simulink model "S7_Legacy_HotStart_Average_Plant"  (R2024b)
settings: Solver=ode15s  StartTime=0.0  StopTime=10  FixedStep=4e-6  MaxStep=1e-4  RelTol=1e-5  EnableMultiTasking=on
InitFcn:
  | s7SourceDir='D:\博士工作\论文工作\（1）构网型风电机组\构网型风电机组\5MW_Ideal\CurrentModel_Idealized';
  | dtime=4e-6;
  | Ts_step=1e-6;
  | run(fullfile(s7SourceDir,'TwoMass_Stage4_Params_5MW_Liu2024.m'));
  | run(fullfile(s7SourceDir,'TwoMass_Working_Experiment_Params.m'));
  | % Default disabled Vdc-reference profile interface (5 MW).
  | if ~exist('Vdc_ref_profile_keep','var') || ~Vdc_ref_profile_keep
  |     Vdc_ref_profile_ts = timeseries([1500;1500],[0;1e6]);
  | end
  | % IdealAvg copy-only electrical network sample time.
  | Ts_step=4e-6;
  | 
  | run(fullfile(s7SourceDir,'initialize_currentmodel_continuous_controller.m'));
  | addpath('D:\博士工作\论文工作\（1）构网型风电机组\构网型风电机组\5MW_Ideal\M3_Workpoint_Generalization\temp\S7_5_LegacyPlant');
  | IdealCfIabc0=-IdealCfIabc0; % S7 hot-start SPS damping-branch orientation correction
  | IdealCfVabc0=IdealCfVabc0+[9.162; -2.039; -7.122]; % S7 hot-start PCC measurement-plane correction
  | addpath('D:\博士工作\论文工作\（1）构网型风电机组\构网型风电机组\5MW_Ideal\M3_Workpoint_Generalization\temp\S7_5_LegacyPlant');
  | hotCfgFile='D:\博士工作\论文工作\（1）构网型风电机组\构网型风电机组\5MW_Ideal\M3_Workpoint_Generalization\temp\S7_5_LegacyPlant\S7_Legacy_HotStart_Config.mat'; hotCfg=load(hotCfgFile,'hotstart_vector','hotstart_vref_V'); S7_LegacyHotStartVector=hotCfg.hotstart_vector; S7_LegacyHotStartVref=hotCfg.hotstart_vref_V;
undefined symbols (not defined in the file): aero_release_delay_s, air_density, cp_beta_bp, cp_lambda_bp, cp_table, D_aero, D_sh, grid_frequency_hz, grid_voltage_peak_V, IdealCtrlPVec, IdealGSCAlpha0, IdealGSCBeta0, IdealLfIabc0, IdealLgIabc0, IdealMSCAlpha0, IdealMSCBeta0, IdealPmsgId0, IdealPmsgIq0, J_g, J_t, K_opt, K_sh, mppt_rated_blend_high_pu, mppt_rated_blend_low_pu, omega_m0, P_wt_rated, pitch_beta_ff_gain_deg_per_mps, pitch_beta_max_deg, pitch_enable, pitch_ff_start_wind_speed, pitch_integrator_initial_deg, pitch_ki_deg_per_rad, pitch_kp_deg_per_radps, pitch_rate_deg_per_s, rated_power_transition_duration_s, rated_power_transition_start_s, rotor_area, rotor_radius, stage4_aero_speed_damping_scale, stage4_ramp_duration_s, stage4_start_s, stage4_torque_ramp_Nmps, theta_tw_stage4_0, v_w0
libraries: spsCurrentMeasurementLib x12, spsSeriesRLCBranchLib x9, spsControlledVoltageSourceLib x6, spsVoltageMeasurementLib x6, simulink x3, powerlib_extras x2, spsControlledCurrentSourceLib x2, spsGroundLib x1, spsThreePhaseSourceLib x1, spsThreePhaseBreakerLib x1, sps_lib x1
(part 2 of 2)

== system S7_Legacy_HotStart_Average_Plant/PMSM1/PMComponent/CURRENT INJECTION SYSTEM ==
  currents : Inport
  Controlled Current Source : spsControlledCurrentSourceLib/Controlled Current Source  Initialize=on  Source_Type=AC  Amplitude=0  Phase=0  Frequency=0  Measurements=None
  Controlled Current Source1 : spsControlledCurrentSourceLib/Controlled Current Source  Initialize=on  Source_Type=AC  Amplitude=0  Phase=0  Frequency=0  Measurements=None
  Demux : Demux  Outputs=2
  Selector : Selector  InputPortWidth=3  IndexOptions=Index vector (dialog)  Indices=1:2  OutputSizes=1
  A1 : PMIOPort  Side=Right
  B1 : PMIOPort  Port=2  Side=Right
  C1 : PMIOPort  Port=3  Side=Right
  wires:
  Demux/1 -> Controlled Current Source/1
  Demux/2 -> Controlled Current Source1/1
  currents/1 -> Selector/1
  Selector/1 -> Demux/1
  connections:
  Controlled Current Source/LConn1 -- A1/RConn1
  Controlled Current Source1/LConn1 -- B1/RConn1
  Controlled Current Source/RConn1 -- Controlled Current Source1/RConn1 -- C1/RConn1

== system S7_Legacy_HotStart_Average_Plant/PMSM1/PMComponent/MEASUREMENT SYSTEM ==
  Mux : Mux  Inputs=3
  V_AB : spsVoltageMeasurementLib/Voltage Measurement  PhasorSimulation=off  OutputType=Complex  PSBequivalent=0
  V_BC : spsVoltageMeasurementLib/Voltage Measurement  PhasorSimulation=off  OutputType=Complex  PSBequivalent=0
  V_CA : spsVoltageMeasurementLib/Voltage Measurement  PhasorSimulation=off  OutputType=Complex  PSBequivalent=0
  A1 : PMIOPort  Side=Left
  B1 : PMIOPort  Port=2  Side=Left
  C1 : PMIOPort  Port=3  Side=Left
  u_line : Outport
  wires:
  Mux/1 -> u_line/1
  V_BC/1 -> Mux/2
  V_AB/1 -> Mux/1
  V_CA/1 -> Mux/3
  connections:
  V_AB/LConn1 -- A1/RConn1 -- V_CA/LConn2
  V_BC/LConn2 -- C1/RConn1 -- V_CA/LConn1
  V_BC/LConn1 -- V_AB/LConn2 -- B1/RConn1

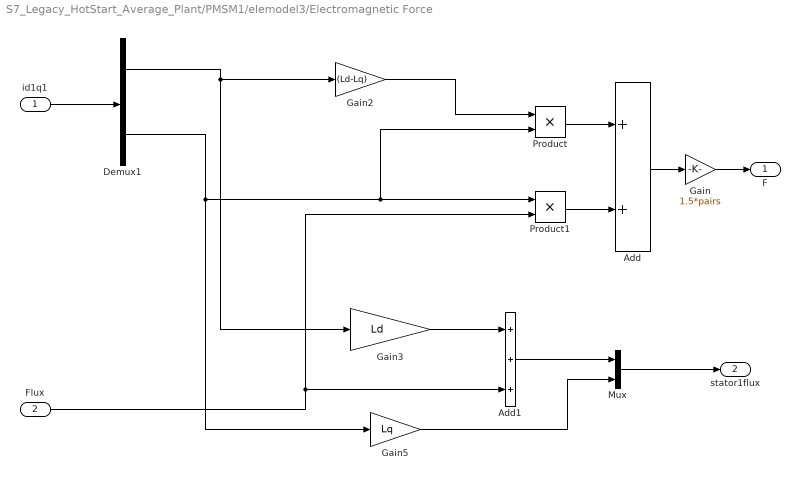
== system S7_Legacy_HotStart_Average_Plant/PMSM1/elemodel3/Electromagnetic Force ==
  id1q1 : Inport
  Flux : Inport  Port=2
  Add : Sum
  Add1 : Sum  Inputs=+++
  Demux1 : Demux  Outputs=2
  Gain : Gain  Gain=1.5*pairs
  Gain2 : Gain  Gain=(Ld-Lq)
  Gain3 : Gain  Gain=Ld
  Gain5 : Gain  Gain=Lq
  Mux : Mux  Inputs=2
  Product : Product  RndMeth=Zero
  Product1 : Product  RndMeth=Zero
  F : Outport
  stator1flux : Outport  Port=2
  wires:
  id1q1/1 -> Demux1/1
  Add/1 -> Gain/1
  Product/1 -> Add/1
  Product1/1 -> Add/2
  Gain/1 -> F/1
  Gain3/1 -> Add1/1
  Add1/1 -> Mux/1
  Mux/1 -> stator1flux/1
  Flux/1 -> Product1/2, Add1/3
  Demux1/2 -> Product1/1, Product/2, Gain5/1
  Demux1/1 -> Gain2/1, Gain3/1
  Gain2/1 -> Product/1
  Gain5/1 -> Mux/2

== system S7_Legacy_HotStart_Average_Plant/PMSM1/elemodel3/abc to dq ==
  uline : Inport
  sin,cos : Inport  Port=2
  Demux : Demux  Outputs=2
  Demux1 : Demux  Outputs=2
  Mux : Mux
  Stationary reference frame : Subsystem  AncestorBlock="spsAsynchronousMachineModel/Continuous/abc to dq  transformation/Stationary reference frame"  TreatAsAtomicUnit=on
      mask Display: disp('Stationary\nreference\nframe')
  linetophase : Subsystem
  statorvoltage : Outport
  V_dq1 : Outport  Port=2
  wires:
  uline/1 -> linetophase/1(v_line)
  Stationary reference frame/1(V_dq) -> V_dq1/1
  linetophase/2(v_alfabeta) -> Demux/1
  sin,cos/1 -> Demux1/1
  Demux/1 -> Mux/1
  Demux/2 -> Mux/2
  Demux1/1 -> Mux/3
  Demux1/2 -> Mux/4
  Mux/1 -> Stationary reference frame/1(ab)
  linetophase/1(stator_voltage) -> statorvoltage/1

== system S7_Legacy_HotStart_Average_Plant/PMSM1/elemodel3/dqtoabc ==
  sincos : Inport
  dq : Inport  Port=2
  Mux : Mux  Inputs=2
  Mux1 : Mux  Inputs=2
  Mux2 : Mux  Inputs=3
  a : Fcn  Expr=u(1)
  alfa : Fcn  Expr=u(1)*u(4)-u(2)*u(3)
  b : Fcn  Expr=(-0.5*u(1)+sqrt(3)*u(2)/2)
  beta : Fcn  Expr=u(1)*u(3)+u(2)*u(4)
  c : Fcn  Expr=(-0.5*u(1)-sqrt(3)*u(2)/2)
  abc : Outport
  wires:
  Mux/1 -> alfa/1, beta/1
  alfa/1 -> Mux1/1
  beta/1 -> Mux1/2
  Mux1/1 -> a/1, b/1, c/1
  a/1 -> Mux2/1
  b/1 -> Mux2/2
  c/1 -> Mux2/3
  dq/1 -> Mux/1
  sincos/1 -> Mux/2
  Mux2/1 -> abc/1

== system S7_Legacy_HotStart_Average_Plant/PMSM1/elemodel3/iq,id ==
  vd1,vq1 : Inport
  we : Inport  Port=2
  Flux : Inport  Port=3
  Demux : Demux  Outputs=2
  Mux : Mux  Inputs=2
  id : Subsystem
  iq : Subsystem
  id1,iq1 : Outport  InitialOutput=0
  wires:
  Mux/1 -> id1,iq1/1
  vd1,vq1/1 -> Demux/1
  Demux/1 -> id/1(vd1)
  Demux/2 -> iq/3(vq)
  id/1(id) -> iq/1(id), Mux/1
  we/1 -> iq/2(we), id/2(we)
  iq/1(iq) -> id/3(iq1), Mux/2
  Flux/1 -> iq/4(Flux)

== system S7_Legacy_HotStart_Average_Plant/PMSM1/elemodel3/sin(thr),cos(thr)1 ==
  thr : Inport
  Mux2 : Mux  Inputs=2
  Trigonometric Function : Trigonometry
  Trigonometric Function1 : Trigonometry  Operator=cos
  sin(thr),cos(thr) : Outport  OutputWhenDisabled=reset  InitialOutput=0
  wires:
  thr/1 -> Trigonometric Function1/1, Trigonometric Function/1  "thr"
  Mux2/1 -> sin(thr),cos(thr)/1
  Trigonometric Function1/1 -> Mux2/2
  Trigonometric Function/1 -> Mux2/1

== system S7_Legacy_HotStart_Average_Plant/PMSM1/elemodel3/abc to dq/Stationary reference frame ==
  ab : Inport
  Mux3 : Mux  Inputs=2
  d : Fcn  Expr=u(4)*u(1)+u(3)*u(2)
  q : Fcn  Expr=-u(3)*u(1)+u(4)*u(2)
  V_dq : Outport  OutputWhenDisabled=reset  InitialOutput=0
  wires:
  d/1 -> Mux3/1
  q/1 -> Mux3/2
  ab/1 -> d/1, q/1
  Mux3/1 -> V_dq/1
  ? -> ?

== system S7_Legacy_HotStart_Average_Plant/PMSM1/elemodel3/abc to dq/linetophase ==
  v_line : Inport
  Mux1 : Mux  Inputs=2
  Mux2 : Mux  Inputs=3
  a : Fcn  Expr=-(u(3)-u(1))/3
  alpha : Fcn  Expr=(2/3)*(u(1)-0.5*u(2)-0.5*u(3))
  b : Fcn  Expr=-(u(1)-u(2))/3
  beta : Fcn  Expr=(2/3)*(sqrt(3)*u(2)/2-sqrt(3)*u(3)/2)
  c : Fcn  Expr=-(u(2)-u(3))/3
  stator_voltage : Outport
  v_alfabeta : Outport  Port=2
  wires:
  a/1 -> Mux2/1
  b/1 -> Mux2/2
  c/1 -> Mux2/3
  v_line/1 -> b/1, a/1, c/1
  Mux2/1 -> beta/1, alpha/1, stator_voltage/1
  alpha/1 -> Mux1/1
  beta/1 -> Mux1/2
  Mux1/1 -> v_alfabeta/1

== system S7_Legacy_HotStart_Average_Plant/PMSM1/elemodel3/iq,id/id ==
  vd1 : Inport
  we : Inport  Port=2
  iq1 : Inport  Port=3
  1/Ld : Gain  Gain=1/Ld  SaturateOnIntegerOverflow=on  OutDataTypeStr=Inherit: Same as input  ParamDataTypeStr=Inherit: Same as input
  Discrete-Time Integrator : Integrator  InitialCondition=IdealPmsgId0
  Lq/Ld : Gain  Gain=Lq/Ld  SaturateOnIntegerOverflow=on  OutDataTypeStr=Inherit: Same as input  ParamDataTypeStr=Inherit: Same as input
  Product1 : Product  InputSameDT=on  SaturateOnIntegerOverflow=on  OutDataTypeStr=Inherit: Same as first input
  R/Ld : Gain  Gain=Rs/Ld  SaturateOnIntegerOverflow=on  OutDataTypeStr=Inherit: Same as input  ParamDataTypeStr=Inherit: Same as input
  Sum1 : Sum  Inputs=-++  InputSameDT=on  SaturateOnIntegerOverflow=on  OutDataTypeStr=Inherit: Same as first input
  id : Outport  InitialOutput=0
  wires:
  R/Ld/1 -> Sum1/1
  Product1/1 -> Lq/Ld/1
  iq1/1 -> Product1/1
  vd1/1 -> 1/Ld/1
  we/1 -> Product1/2
  Lq/Ld/1 -> Sum1/2
  1/Ld/1 -> Sum1/3
  Sum1/1 -> Discrete-Time Integrator/1
  Discrete-Time Integrator/1 -> id/1, R/Ld/1

== system S7_Legacy_HotStart_Average_Plant/PMSM1/elemodel3/iq,id/iq ==
  id : Inport
  we : Inport  Port=2
  vq : Inport  Port=3
  Flux : Inport  Port=4
  1/Lq : Gain  Gain=1/Lq  SaturateOnIntegerOverflow=on  OutDataTypeStr=Inherit: Same as input  ParamDataTypeStr=Inherit: Same as input
  1/Lq1 : Gain  Gain=1/Lq  SaturateOnIntegerOverflow=on  OutDataTypeStr=Inherit: Same as input  ParamDataTypeStr=Inherit: Same as input
  Discrete-Time Integrator : Integrator  InitialCondition=IdealPmsgIq0
  Ld1/Lq1 : Gain  Gain=Ld/Lq  SaturateOnIntegerOverflow=on  OutDataTypeStr=Inherit: Same as input  ParamDataTypeStr=Inherit: Same as input
  Product : Product  InputSameDT=on  SaturateOnIntegerOverflow=on  OutDataTypeStr=Inherit: Same as first input
  Product1 : Product  InputSameDT=on  SaturateOnIntegerOverflow=on  OutDataTypeStr=Inherit: Same as first input
  R/Lq : Gain  Gain=Rs/Lq  SaturateOnIntegerOverflow=on  OutDataTypeStr=Inherit: Same as input  ParamDataTypeStr=Inherit: Same as input
  Sum : Sum  Inputs=-+--  InputSameDT=on  SaturateOnIntegerOverflow=on  OutDataTypeStr=Inherit: Same as first input
  iq : Outport  InitialOutput=0
  wires:
  R/Lq/1 -> Sum/1
  Product/1 -> Ld1/Lq1/1
  vq/1 -> 1/Lq/1
  we/1 -> Product/1, Product1/1
  id/1 -> Product/2
  Product1/1 -> 1/Lq1/1
  Flux/1 -> Product1/2
  1/Lq/1 -> Sum/2
  Ld1/Lq1/1 -> Sum/3
  1/Lq1/1 -> Sum/4
  Sum/1 -> Discrete-Time Integrator/1
  Discrete-Time Integrator/1 -> iq/1, R/Lq/1
